simulink model "RailP"  (R2018a)
settings: configuration reference "cs_ert" (kept outside this file)
settings Model: DataDictionary=RailP.sldd  Creator=zhoutinglin  LastModifiedBy=zhoutinglin

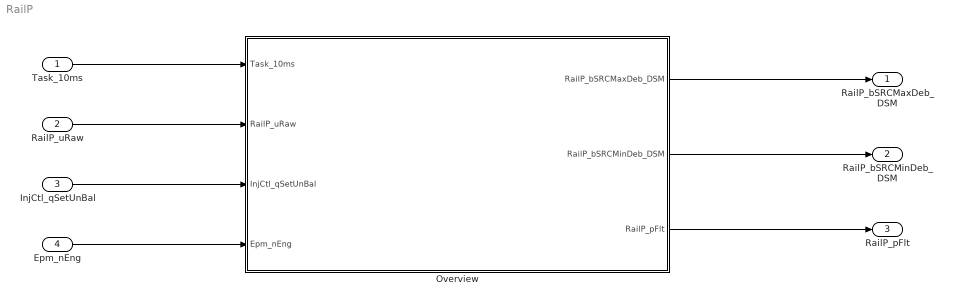
== system RailP ==
  Task_10ms : Inport  OutputFunctionCall=on
  RailP_uRaw : Inport  Port=2
  InjCtl_qSetUnBal : Inport  Port=3
  Epm_nEng : Inport  Port=4
  Overview : Subsystem
  RailP_bSRCMaxDeb_DSM : Outport
  RailP_bSRCMinDeb_DSM : Outport  Port=2
  RailP_pFlt : Outport  Port=3
  wires:
  Task_10ms/1 -> Overview/1(Task_10ms)
  RailP_uRaw/1 -> Overview/2(RailP_uRaw)
  InjCtl_qSetUnBal/1 -> Overview/3(InjCtl_qSetUnBal)
  Epm_nEng/1 -> Overview/4(Epm_nEng)
  Overview/1(RailP_bSRCMaxDeb_DSM) -> RailP_bSRCMaxDeb_DSM/1
  Overview/2(RailP_bSRCMinDeb_DSM) -> RailP_bSRCMinDeb_DSM/1
  Overview/3(RailP_pFlt) -> RailP_pFlt/1

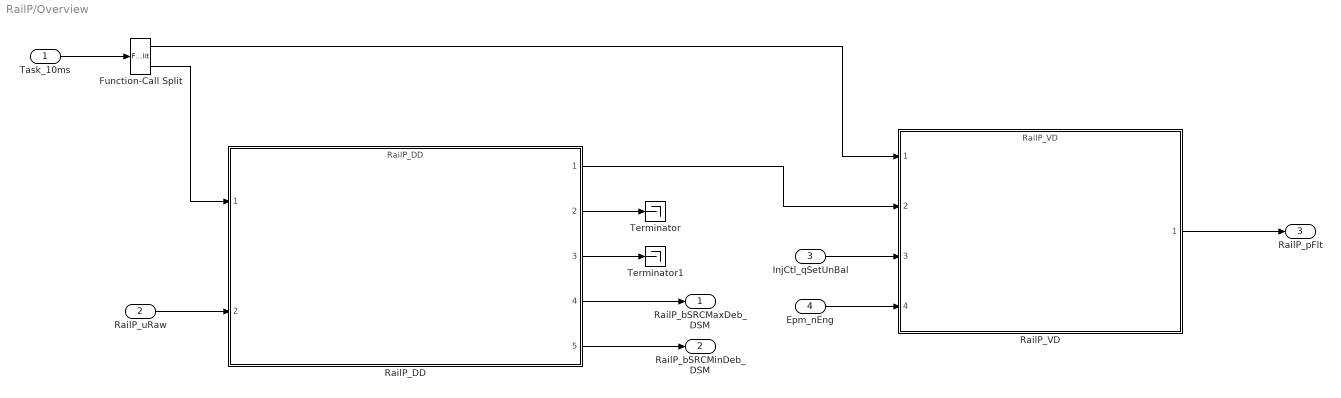
== system RailP/Overview ==
  Task_10ms : Inport
  RailP_uRaw : Inport  Port=2
  InjCtl_qSetUnBal : Inport  Port=3
  Epm_nEng : Inport  Port=4
  Function-Call Split : FunctionCallSplit  IconShape=distinctive  NumOutputPorts=2  OutputPortLayout=default
  RailP_DD : ModelReference  ModelNameDialog=RailP_DD  SimulationMode=Normal  ModelReferenceVersion=1.55
  RailP_VD : ModelReference  ModelNameDialog=RailP_VD  SimulationMode=Normal  ModelReferenceVersion=1.53
  Terminator : Terminator
  Terminator1 : Terminator
  RailP_bSRCMaxDeb_DSM : Outport
  RailP_bSRCMinDeb_DSM : Outport  Port=2
  RailP_pFlt : Outport  Port=3
  wires:
  RailP_DD/4 -> RailP_bSRCMaxDeb_DSM/1
  RailP_DD/5 -> RailP_bSRCMinDeb_DSM/1
  RailP_VD/1 -> RailP_pFlt/1
  RailP_DD/2 -> Terminator/1
  RailP_DD/3 -> Terminator1/1
  RailP_uRaw/1 -> RailP_DD/2
  RailP_DD/1 -> RailP_VD/2
  InjCtl_qSetUnBal/1 -> RailP_VD/3
  Epm_nEng/1 -> RailP_VD/4
  Task_10ms/1 -> Function-Call Split/1
  Function-Call Split/2 -> RailP_DD/1
  Function-Call Split/1 -> RailP_VD/1
